simulink model "WMMSupportingForcesGP2020a"  (R2020a)
settings: Solver=ode23t  StartTime=0.0  StopTime=inf  FixedStep=.001  RelTol=1e-3  AbsTol=1e-3
InitFcn:
  | InitializeSimulationGP
  | SimulationParametersGP
values from neighbouring files (symbols this model uses):
  B11_r_B11C = [0.23805608; 0.13201777; 0]    [InitializeSimulationGP.m]
  B11_r_B11Tc1 = [L11; 0; 0]    [InitializeSimulationGP.m]
  B11_Rot_Tc1 = eye(3)    [InitializeSimulationGP.m]
  B11cI = [0.28426000 -0.06487287 0;         -0.06487287  0.54237481 0;                   0  0          0.67891020]    [InitializeSimulationGP.m]
  B12_r_B12C = [0.60504569; 0.27199376; 0.00002484]    [InitializeSimulationGP.m]
  B12_r_B12Tc2 = [L12;0;0]    [InitializeSimulationGP.m]
  B12_Rot_Tc2 = eye(3)    [InitializeSimulationGP.m]
  B12cI = [1.18803886 -2.36786418 0.00280315;          -2.36786418 6.31493281 0.00022322;           0.00280315 0.00022322 7.40915161]    [InitializeSimulationGP.m]
  B31_r_B31C = [0.35781210 0 0]    [InitializeSimulationGP.m]
  B31_Rot_B41 = eye(3)    [InitializeSimulationGP.m]
  B31cI = diag([0.03150902 0.90735702 0.90763033])    [InitializeSimulationGP.m]
  B32_r_B32C = [0.35781210 0 0]    [InitializeSimulationGP.m]
  B32_Rot_B42 = eye(3)    [InitializeSimulationGP.m]
  B32cI = diag([0.03150902 0.90735702 0.90763033])    [InitializeSimulationGP.m]
  B41_r_B41C = [0.55785997 0 0]    [InitializeSimulationGP.m]
  B41_r_B41Tc1 = [lc1;0;0]    [InitializeSimulationGP.m]
  B41cI = diag([0.00370720 0.55759812 0.55785997])    [InitializeSimulationGP.m]
  B42_r_B42C = [0.55785997 0 0]    [InitializeSimulationGP.m]
  B42_r_B42Tc2 = [lc2; 0; 0]    [InitializeSimulationGP.m]
  B42cI = diag([0.00370720 0.55759812 0.55785997])    [InitializeSimulationGP.m]
  B52_r_B52C = [0 0 0.56802906]    [InitializeSimulationGP.m]
  B52_r_B52P32 = [lc3; 0; 0]    [InitializeSimulationGP.m]
  B52_Rot_P32 = eye(3)    [InitializeSimulationGP.m]
  B52cI = diag([0.91789884, 0.91790043, 0.00091463])    [InitializeSimulationGP.m]
  Bc1_r_Bc1B11 = [L1; 0; 0]    [InitializeSimulationGP.m]
  Bc1_r_Bc1B31 = [0;0;0]    [InitializeSimulationGP.m]
  Bc1_r_Bc1C = [0.14178771; 0.16555780; 0]    [InitializeSimulationGP.m]
  Bc1_V = [0;0;0;0;0;0]    [InitializeSimulationGP.m]
  Bc1cI = [+5.892211080 +5.476111360 -0.000019630;          +5.476111360 +28.66965601 -0.000024550;          -0.000019630 -0.000024550 +29.78955950]    [InitializeSimulationGP.m]
  Bc2_r_Bc2B12 = [L2;0;0]    [InitializeSimulationGP.m]
  Bc2_r_Bc2B32 = [0;0;0]    [InitializeSimulationGP.m]
  Bc2_r_Bc2C = [0.54319901; 0.10543875; 0]    [InitializeSimulationGP.m]
  Bc2cI = [0.48071390 0.52924041 0;          0.52924041 5.80912352 0;              0      0          5.97255351]    [InitializeSimulationGP.m]
  BC_r_BCBM = [xCA; yCA; zCA]    [SimulationParametersGP.m]
  BC_Rot_BM = eye(3)    [SimulationParametersGP.m]
  BCI = diag([100 1200 1000])    [SimulationParametersGP.m]
  beta1 = atan2d(374.261,935)*pi/180    [InitializeSimulationGP.m]
  beta2 = atan2d(45.757,373.313)*pi/180    [InitializeSimulationGP.m]
  beta3 = atan2d(139.50,1132.19)*pi/180    [InitializeSimulationGP.m]
  beta4 = atan2d(88.061,296.198)*pi/180    [InitializeSimulationGP.m]
  betaGround = 1e6    (= 1000000)    [SimulationParametersGP.m]
  BFL = 0.05    [SimulationParametersGP.m]
  BFR = 0.05    [SimulationParametersGP.m]
  BM_r_BMBMp = [0;0;0]    [SimulationParametersGP.m]
  BM_Rot_BMp = [cos(gamma) -sin(gamma) 0; sin(gamma) cos(gamma) 0; 0 0 1]    [SimulationParametersGP.m]
  BMp_r_BMpBc1 = [0.185;0;0.205]    [InitializeSimulationGP.m]
  BMp_Rot_Bc1 = [cos(alpha1) -sin(alpha1)  0;                  0            0       -1;                sin(alpha1)  cos(alpha1)  0]    [InitializeSimulationGP.m]
  BRL = 0.05    [SimulationParametersGP.m]
  BRR = 0.05    [SimulationParametersGP.m]
  cc = 0.0    (= 0)    [SimulationParametersGP.m]
  D22F = [0;0;0;0;0;0]    [InitializeSimulationGP.m]
  dT = 0.01    [SimulationParametersGP.m]
  g0 = 9.8066    [SimulationParametersGP.m]
  ground_stiffness = 1e8    (= 100000000)    [SimulationParametersGP.m]
  l1 = 1.15-cc    (= 1.15)    [SimulationParametersGP.m]
  L1 = 1.0071227324212    (= 1.00712273242)    [InitializeSimulationGP.m]
  L11 = 0.37610632101293    (= 0.376106321013)    [InitializeSimulationGP.m]
  L12 = 0.30901132665325    (= 0.309011326653)    [InitializeSimulationGP.m]
  l2 = 1.15+cc    (= 1.15)    [SimulationParametersGP.m]
  L2 = 1.132185817991    (= 1.13218581799)    [InitializeSimulationGP.m]
  lc1 = 0.745    [InitializeSimulationGP.m]
  lc2 = 0.745    [InitializeSimulationGP.m]
  mB11 = 25.52660174    [InitializeSimulationGP.m]
  mB12 = 33.92850233    [InitializeSimulationGP.m]
  mB31 = 17.36281648    [InitializeSimulationGP.m]
  mB32 = 17.36281648    [InitializeSimulationGP.m]
  mB41 = 10.34519231    [InitializeSimulationGP.m]
  mB42 = 10.34519231    [InitializeSimulationGP.m]
  mB52 = 6.73059863    [InitializeSimulationGP.m]
  mBC = 2200    [SimulationParametersGP.m]
  mBc1 = 307.29601379    [InitializeSimulationGP.m]
  mBc2 = 54.58702836    [InitializeSimulationGP.m]
  mFL = 60    [SimulationParametersGP.m]
  mFR = 60    [SimulationParametersGP.m]
  mP22 = 9.26136143    [InitializeSimulationGP.m]
  mP32 = 570.18877059    [InitializeSimulationGP.m]
  mRR = 60    [SimulationParametersGP.m]
  mw = mFL    (= 60)    [SimulationParametersGP.m]
  P22_r_P22C = [0.62192523 0 0]    [InitializeSimulationGP.m]
  P22_Rot_B52 = eye(3)    [InitializeSimulationGP.m]
  P22cI = diag([0.00662754, 1.48387017, 1.48398069])    [InitializeSimulationGP.m]
  P32_r_P32C = [0.25466704; -0.13034397; -0.01302248]    [InitializeSimulationGP.m]
  P32_r_P32D22 = [0.40499744871392; -0.13130517281345; -0.013385243295654]    [InitializeSimulationGP.m]
  P32_Rot_D22 = [1 0 0;              0 0.9707729441837 0.23999977258512;              0 -0.23999977258512 0.9707729441837]    [InitializeSimulationGP.m]
  P32cI = [46.81220713 0.38607676 -0.00453819;          0.38607676 71.92201786 -1.14320993;          -0.00453819 -1.14320993 67.38128576]    [InitializeSimulationGP.m]
  R0FL = 0.35    [SimulationParametersGP.m]
  R0FR = 0.35    [SimulationParametersGP.m]
  R0RL = 0.35    [SimulationParametersGP.m]
  R0RR = 0.35    [SimulationParametersGP.m]
  Rw = R0FL    (= 0.35)    [SimulationParametersGP.m]
  Tc1_r_Tc1Bc2 = [0.098495302558553; 0.01838181329939; 0]    [InitializeSimulationGP.m]
  Tc1_Rot_Bc2 = [cos(alpha2) -sin(alpha2) 0;                sin(alpha2)  cos(alpha2) 0;                0            0           1]    [InitializeSimulationGP.m]
  Tc2_r_Tc2P22 = [-0.048858374920227;0.36587359346146;0.035276938723102]    [InitializeSimulationGP.m]
  Tc2_Rot_P22 = [0.95853460763586 -0.27664713597974  0.0683942111482;                0.28497614981675  0.93051946315663 -0.23004808784757;                0                 0.23999977258511  0.9707729441837]    [InitializeSimulationGP.m]
  Th1A = 10*pi/180    (= 0.174532925199)    [InitializeSimulationGP.m]
  Th1B = 20*pi/180    (= 0.349065850399)    [InitializeSimulationGP.m]
  Th1f = 1    [InitializeSimulationGP.m]
  Th2A = 15*pi/180    (= 0.261799387799)    [InitializeSimulationGP.m]
  Th2B = -70*pi/180    (= -1.2217304764)    [InitializeSimulationGP.m]
  Th2f = 2    [InitializeSimulationGP.m]
  w = wFL    (= 0.875)    [SimulationParametersGP.m]
  W_r_WBc1 = [0.185;0;0.205]    [InitializeSimulationGP.m]
  W_Rot_Bc1 = [cos(alpha1) -sin(alpha1)  0;                  0            0       -1;                sin(alpha1)  cos(alpha1)  0]    [InitializeSimulationGP.m]
  x10 = 0.83    [InitializeSimulationGP.m]
  x20 = 0.83    [InitializeSimulationGP.m]
  x3A = 0.2    [InitializeSimulationGP.m]
  x3B = 0.3    [InitializeSimulationGP.m]
  x3f = 1    [InitializeSimulationGP.m]
  xCA = 0.5    [SimulationParametersGP.m]
  xf = [1;0;0;0;0;0]    [InitializeSimulationGP.m]
  yCA = 0    [SimulationParametersGP.m]
  zC = 0.45    [SimulationParametersGP.m]
  zCA = .25    (= 0.25)    [SimulationParametersGP.m]
  ztau = [0;0;0;0;0;1]    [InitializeSimulationGP.m]
undefined symbols (not defined in the file or in its folder): alphaFL_meas, alphaFR_meas, alphaRL_meas, alphaRR_meas, B11_V, B11Ftot, B12_U_Tc2, B12_V, B12Ftot, B31_r_B31B41, B31_V, B31FTot, B32_r_B32B42, B32_U_B42, B32_V, B32FTot, B41_V, B41FTot, B42_Rot_Tc2, B42_U_Tc2, B42_V, B42FTot, B52_U_P32, B52_V, B52Ftot, Bc1Tot, Bc2_Rot_B12, Bc2_Rot_B32, Bc2_U_B12, Bc2_U_B32, Bc2_V, Bc2Tot, betaC_meas, D22_V, deltaFL_cmd, deltaFL_meas, deltaFR_cmd, deltaFR_meas, deltaRL_cmd, deltaRL_meas, deltaRR_cmd, deltaRR_meas, dOmegaFL_meas, dOmegaFR_meas, dOmegaRL_meas, dOmegaRR_meas, dPsi_meas, dq1, dq11, dq12, dq2, dq21, dq22, dx1, dx2, Floor, FTot_S1, FTot_S2P, FTot_S2R, FzFL ... (+63)
libraries: sm_lib x94, nesl_utility x63, simulink x5
(part 11 of 11)

== matlab function WMMSupportingForcesGP2020a/calc_wheel_velocities_and_sideslip_angles_from_meas/Hydraulic manipulator, calculation/AnalyticTotalForces/Structure 2 (Prismatic segment)/MATLAB Function2 ==
  data: B52V input; B52a input; B52w input; B52dw input; B52_Rot_W input; Wg parameter; YB52 output
function YB52  = thetaB52(B52V, B52a, B52w, B52dw, B52_Rot_W,  Wg)

vx = B52V(1);
vy = B52V(2);
vz = B52V(3);
ax = B52a(1);
ay = B52a(2);
az = B52a(3);
wx = B52w(1);
wy = B52w(2);
wz = B52w(3);
dwx = B52dw(1);
dwy = B52dw(2);
dwz = B52dw(3);
B52g = B52_Rot_W*Wg;
gx = B52g(1);
gy = B52g(2);
gz = B52g(3);

Y11 = ( ax + vz * wy - vy * wz  + gx);
t5 = (wy *  wy);
t6 = (wz * wz);
Y12 = -t5 - t6;
t7 = (wx * wy);
Y13 = (t7 - dwz);
t8 = (wx * wz);
Y14 = (t8 + dwy);
Y15 = 0;
Y16 = 0;
Y17 = 0;
Y18 = 0;
Y19 = 0;
Y110 = 0;
Y111 = 0;
Y112 = 0;
Y113 = 0;
Y21 = vx * wz - vz * wx + ay + gy;
Y22 = t7 + dwz;
t11 = wx * wx;
Y23 = -t11 - t6;
t12 = wy * wz;
Y24 = t12 - dwx;
Y25 = 0;
Y26 = 0;
Y27 = 0;
Y28 = 0;
Y29 = 0;
Y210 = 0;
Y211 = 0;
Y212 = 0;
Y213 = 0;
Y31 = -vx * wy + vy * wx + az + gz;
Y32 = t8 - dwy;
Y33 = t12 + dwx;
Y34 = -t11 - t5;
Y35 = 0;
Y36 = 0;
Y37 = 0;
Y38 = 0;
Y39 = 0;
Y310 = 0;
Y311 = 0;
Y312 = 0;
Y313 = 0;
Y41 = 0;
Y42 = 0;
Y43 = Y31;
Y44 = -Y21;
Y45 = 0;
Y46 = Y33;
Y47 = -Y24;
Y48 = Y32;
Y49 = -Y22;
Y410 = -t5 + t6;
Y411 = dwx;
Y412 = -t12;
Y413 = t12;
Y51 = 0;
Y52 = -Y31;
Y53 = 0;
Y54 = Y11;
Y55 = -Y32;
Y56 = 0;
Y57 = Y14;
Y58 = -Y33;
Y59 = t11 - t6;
Y510 = Y13;
Y511 = t8;
Y512 = dwy;
Y513 = -t8;
Y61 = 0;
Y62 = Y21;
Y63 = -Y11;
Y64 = 0;
Y65 = Y22;
Y66 = -Y13;
Y67 = 0;
Y68 = t5 - t11;
Y69 = Y24;
Y610 = -Y14;
Y611 = -t7;
Y612 = t7;
Y613 = dwz;

YB52 = [Y11 Y12 Y13 Y14 Y15 Y16 Y17 Y18 Y19 Y110 Y111 Y112 Y113;...
        Y21 Y22 Y23 Y24 Y25 Y26 Y27 Y28 Y29 Y210 Y211 Y212 Y213;...
        Y31 Y32 Y33 Y34 Y35 Y36 Y37 Y38 Y39 Y310 Y311 Y312 Y313;...
        Y41 Y42 Y43 Y44 Y45 Y46 Y47 Y48 Y49 Y410 Y411 Y412 Y413;...
        Y51 Y52 Y53 Y54 Y55 Y56 Y57 Y58 Y59 Y510 Y511 Y512 Y513;...
        Y61 Y62 Y63 Y64 Y65 Y66 Y67 Y68 Y69 Y610 Y611 Y612 Y613];

== matlab function WMMSupportingForcesGP2020a/calc_wheel_velocities_and_sideslip_angles_from_meas/Hydraulic manipulator, calculation/AnalyticVelocities/Structure 2 (Revolute segment)/RotMatsS2R/B42_Rot_Tc2 ==
  data: q22 input; B42_Rot_Tc2 output
function B42_Rot_Tc2 = B42_Rot_Tc2(q22)

B42_Rot_Tc2 = [+cos(q22) -sin(q22) 0;...
               +sin(q22) +cos(q22) 0;...
                   0        0      1];

== matlab function WMMSupportingForcesGP2020a/calc_wheel_velocities_and_sideslip_angles_from_meas/Hydraulic manipulator, calculation/AnalyticTotalForces/Structure 2 (Prismatic segment)/MATLAB Function3 ==
  data: thetaP32 output; P32_r_P32C parameter; mP32 parameter; P32cI parameter
function thetaP32 = thetaP32(P32_r_P32C, mP32, P32cI)

rx = P32_r_P32C(1);
ry = P32_r_P32C(2);
rz = P32_r_P32C(3);

Ixx = P32cI(1,1);
Iyy = P32cI(2,2);
Izz = P32cI(3,3);
Iyz = P32cI(2,3);
Ixz = P32cI(1,3);
Ixy = P32cI(1,2);

t1 = rx*rx;
t2 = ry*ry;
t3 = rz*rz;
t4 = rx*mP32;

thetaP32 = [mP32; rx*mP32; ry*mP32; rz*mP32; t1*mP32; t2*mP32; t3*mP32; t4*ry - Ixy; t4*rz - Ixz; mP32*ry*rz - Iyz; Ixx; Iyy; Izz];

== matlab function WMMSupportingForcesGP2020a/calc_wheel_velocities_and_sideslip_angles_from_meas/Hydraulic manipulator, calculation/AnalyticTotalForces/Structure 2 (Prismatic segment)/MATLAB Function7 ==
  data: P22V input; P22a input; P22w input; P22dw input; P22_Rot_W input; Wg parameter; YP22 output
function YP22  = thetaP22(P22V, P22a, P22w, P22dw, P22_Rot_W,  Wg)

vx = P22V(1);
vy = P22V(2);
vz = P22V(3);
ax = P22a(1);
ay = P22a(2);
az = P22a(3);
wx = P22w(1);
wy = P22w(2);
wz = P22w(3);
dwx = P22dw(1);
dwy = P22dw(2);
dwz = P22dw(3);
P22g = P22_Rot_W*Wg;
gx = P22g(1);
gy = P22g(2);
gz = P22g(3);

Y11 = ( ax + vz * wy - vy * wz  + gx);
t5 = (wy *  wy);
t6 = (wz * wz);
Y12 = -t5 - t6;
t7 = (wx * wy);
Y13 = (t7 - dwz);
t8 = (wx * wz);
Y14 = (t8 + dwy);
Y15 = 0;
Y16 = 0;
Y17 = 0;
Y18 = 0;
Y19 = 0;
Y110 = 0;
Y111 = 0;
Y112 = 0;
Y113 = 0;
Y21 = vx * wz - vz * wx + ay + gy;
Y22 = t7 + dwz;
t11 = wx * wx;
Y23 = -t11 - t6;
t12 = wy * wz;
Y24 = t12 - dwx;
Y25 = 0;
Y26 = 0;
Y27 = 0;
Y28 = 0;
Y29 = 0;
Y210 = 0;
Y211 = 0;
Y212 = 0;
Y213 = 0;
Y31 = -vx * wy + vy * wx + az + gz;
Y32 = t8 - dwy;
Y33 = t12 + dwx;
Y34 = -t11 - t5;
Y35 = 0;
Y36 = 0;
Y37 = 0;
Y38 = 0;
Y39 = 0;
Y310 = 0;
Y311 = 0;
Y312 = 0;
Y313 = 0;
Y41 = 0;
Y42 = 0;
Y43 = Y31;
Y44 = -Y21;
Y45 = 0;
Y46 = Y33;
Y47 = -Y24;
Y48 = Y32;
Y49 = -Y22;
Y410 = -t5 + t6;
Y411 = dwx;
Y412 = -t12;
Y413 = t12;
Y51 = 0;
Y52 = -Y31;
Y53 = 0;
Y54 = Y11;
Y55 = -Y32;
Y56 = 0;
Y57 = Y14;
Y58 = -Y33;
Y59 = t11 - t6;
Y510 = Y13;
Y511 = t8;
Y512 = dwy;
Y513 = -t8;
Y61 = 0;
Y62 = Y21;
Y63 = -Y11;
Y64 = 0;
Y65 = Y22;
Y66 = -Y13;
Y67 = 0;
Y68 = t5 - t11;
Y69 = Y24;
Y610 = -Y14;
Y611 = -t7;
Y612 = t7;
Y613 = dwz;

YP22 = [Y11 Y12 Y13 Y14 Y15 Y16 Y17 Y18 Y19 Y110 Y111 Y112 Y113;...
        Y21 Y22 Y23 Y24 Y25 Y26 Y27 Y28 Y29 Y210 Y211 Y212 Y213;...
        Y31 Y32 Y33 Y34 Y35 Y36 Y37 Y38 Y39 Y310 Y311 Y312 Y313;...
        Y41 Y42 Y43 Y44 Y45 Y46 Y47 Y48 Y49 Y410 Y411 Y412 Y413;...
        Y51 Y52 Y53 Y54 Y55 Y56 Y57 Y58 Y59 Y510 Y511 Y512 Y513;...
        Y61 Y62 Y63 Y64 Y65 Y66 Y67 Y68 Y69 Y610 Y611 Y612 Y613];

== matlab function WMMSupportingForcesGP2020a/calc_wheel_velocities_and_sideslip_angles_from_meas/Hydraulic manipulator, calculation/AnalyticVelocities/Structure 2 (Revolute segment)/GeomPropS2R/Subsystem4/q21AngularVelocity ==
  data: x2 input; dx2 input; q21 input; dq21 output; L2 parameter; x20 parameter
function dq21 = dq21(x2, dx2, q21, L2, x20)

dq21 = -((x2+x20)-L2*cos(q21))/((x2+x20)*L2*sin(q21))*dx2;

== matlab function WMMSupportingForcesGP2020a/calc_wheel_velocities_and_sideslip_angles_from_meas/Hydraulic manipulator, calculation/AnalyticVelocities/Structure 2 (Revolute segment)/GeomPropS2R/Subsystem5/q22AngularVelocity ==
  data: x2 input; dx2 input; q22 input; dq22 output; L12 parameter; x20 parameter
function dq22 = dq22(x2, dx2, q22, L12, x20)

dq22 = -((x2+x20)-L12*cos(q22))/((x2+x20)*L12*sin(q22))*dx2;

== matlab function WMMSupportingForcesGP2020a/calc_wheel_velocities_and_sideslip_angles_from_meas/Hydraulic manipulator, calculation/AnalyticVelocities/Structure 2 (Revolute segment)/GeomPropS2R/TiltPistonVelocity/TiltPistonVelocity ==
  data: x2 input; q2 input; dq2 input; dx2 output; L2 parameter; L12 parameter; x20 parameter
function dx2 = dx2(x2, q2, dq2, L2, L12, x20)

dx2 = -(L2*L12*sin(q2))/(x2+x20)*dq2;

== matlab function WMMSupportingForcesGP2020a/calc_wheel_velocities_and_sideslip_angles_from_meas/Hydraulic manipulator, calculation/AnalyticTotalForces/Structure 2 (Prismatic segment)/MATLAB Function4 ==
  data: P32V input; P32a input; P32w input; P32dw input; P32_Rot_W input; Wg parameter; YP32 output
function YP32  = thetaP32(P32V, P32a, P32w, P32dw, P32_Rot_W,  Wg)

vx = P32V(1);
vy = P32V(2);
vz = P32V(3);
ax = P32a(1);
ay = P32a(2);
az = P32a(3);
wx = P32w(1);
wy = P32w(2);
wz = P32w(3);
dwx = P32dw(1);
dwy = P32dw(2);
dwz = P32dw(3);
P32g = P32_Rot_W*Wg;
gx = P32g(1);
gy = P32g(2);
gz = P32g(3);

Y11 = ( ax + vz * wy - vy * wz  + gx);
t5 = (wy *  wy);
t6 = (wz * wz);
Y12 = -t5 - t6;
t7 = (wx * wy);
Y13 = (t7 - dwz);
t8 = (wx * wz);
Y14 = (t8 + dwy);
Y15 = 0;
Y16 = 0;
Y17 = 0;
Y18 = 0;
Y19 = 0;
Y110 = 0;
Y111 = 0;
Y112 = 0;
Y113 = 0;
Y21 = vx * wz - vz * wx + ay + gy;
Y22 = t7 + dwz;
t11 = wx * wx;
Y23 = -t11 - t6;
t12 = wy * wz;
Y24 = t12 - dwx;
Y25 = 0;
Y26 = 0;
Y27 = 0;
Y28 = 0;
Y29 = 0;
Y210 = 0;
Y211 = 0;
Y212 = 0;
Y213 = 0;
Y31 = -vx * wy + vy * wx + az + gz;
Y32 = t8 - dwy;
Y33 = t12 + dwx;
Y34 = -t11 - t5;
Y35 = 0;
Y36 = 0;
Y37 = 0;
Y38 = 0;
Y39 = 0;
Y310 = 0;
Y311 = 0;
Y312 = 0;
Y313 = 0;
Y41 = 0;
Y42 = 0;
Y43 = Y31;
Y44 = -Y21;
Y45 = 0;
Y46 = Y33;
Y47 = -Y24;
Y48 = Y32;
Y49 = -Y22;
Y410 = -t5 + t6;
Y411 = dwx;
Y412 = -t12;
Y413 = t12;
Y51 = 0;
Y52 = -Y31;
Y53 = 0;
Y54 = Y11;
Y55 = -Y32;
Y56 = 0;
Y57 = Y14;
Y58 = -Y33;
Y59 = t11 - t6;
Y510 = Y13;
Y511 = t8;
Y512 = dwy;
Y513 = -t8;
Y61 = 0;
Y62 = Y21;
Y63 = -Y11;
Y64 = 0;
Y65 = Y22;
Y66 = -Y13;
Y67 = 0;
Y68 = t5 - t11;
Y69 = Y24;
Y610 = -Y14;
Y611 = -t7;
Y612 = t7;
Y613 = dwz;

YP32 = [Y11 Y12 Y13 Y14 Y15 Y16 Y17 Y18 Y19 Y110 Y111 Y112 Y113;...
        Y21 Y22 Y23 Y24 Y25 Y26 Y27 Y28 Y29 Y210 Y211 Y212 Y213;...
        Y31 Y32 Y33 Y34 Y35 Y36 Y37 Y38 Y39 Y310 Y311 Y312 Y313;...
        Y41 Y42 Y43 Y44 Y45 Y46 Y47 Y48 Y49 Y410 Y411 Y412 Y413;...
        Y51 Y52 Y53 Y54 Y55 Y56 Y57 Y58 Y59 Y510 Y511 Y512 Y513;...
        Y61 Y62 Y63 Y64 Y65 Y66 Y67 Y68 Y69 Y610 Y611 Y612 Y613];

== matlab function WMMSupportingForcesGP2020a/calc_wheel_velocities_and_sideslip_angles_from_meas/Hydraulic manipulator, calculation/AnalyticVelocities/Structure 2 (Revolute segment)/RotMatsS2R/Bc2_Rot_B12 ==
  data: q2 input; Bc2_Rot_B12 output
function Bc2_Rot_B12 = Bc2_Rot_B12(q2)

Bc2_Rot_B12 = [+cos(q2) -sin(q2) 0;...
               +sin(q2) +cos(q2) 0;...
                  0        0     1];

== matlab function WMMSupportingForcesGP2020a/calc_wheel_velocities_and_sideslip_angles_from_meas/Hydraulic manipulator, calculation/AnalyticVelocities/Structure 2 (Revolute segment)/RotMatsS2R/Bc2_Rot_B32 ==
  data: q21 input; Bc2_Rot_B32 output

function Bc2_Rot_B32 = Bc2_Rot_B32(q21)

Bc2_Rot_B32 = [+cos(q21) -sin(q21) 0;...
               +sin(q21) +cos(q21) 0;...
                   0         0     1];

== matlab function WMMSupportingForcesGP2020a/calc_wheel_velocities_and_sideslip_angles_from_meas/Hydraulic manipulator, calculation/AnalyticVelocities/Structure 2 (Revolute segment)/UMatS2R/B12_U_Tc2 ==
  data: B12_r_B12Tc2 input; B12_U_Tc2 output; B12_Rot_Tc2 input
function B12_U_Tc2 = B12_U_Tc2(B12_r_B12Tc2, B12_Rot_Tc2)

B12_U_Tc2 = [B12_Rot_Tc2,                    zeros(3);...
             dual(B12_r_B12Tc2)*B12_Rot_Tc2, B12_Rot_Tc2];
   
end
   
function dual_r = dual(ArAB)

dual_r = [0,  -ArAB(3), ArAB(2);...
          ArAB(3), 0, -ArAB(1);...
          -ArAB(2), ArAB(1), 0];

end

== matlab function WMMSupportingForcesGP2020a/calc_wheel_velocities_and_sideslip_angles_from_meas/Hydraulic manipulator, calculation/AnalyticVelocities/Structure 2 (Revolute segment)/UMatS2R/B32_U_B42 ==
  data: B32_r_B32B42 input; B32_U_B42 output; B32_Rot_B42 input
function B32_U_B42 = B32_U_B42(B32_r_B32B42, B32_Rot_B42)

B32_U_B42 = [B32_Rot_B42,                    zeros(3);...
             dual(B32_r_B32B42)*B32_Rot_B42, B32_Rot_B42];
   
end
   
function dual_r = dual(ArAB)

dual_r = [0,  -ArAB(3), ArAB(2);...
          ArAB(3), 0, -ArAB(1);...
          -ArAB(2), ArAB(1), 0];

end

== matlab function WMMSupportingForcesGP2020a/calc_wheel_velocities_and_sideslip_angles_from_meas/Hydraulic manipulator, calculation/AnalyticVelocities/Structure 2 (Revolute segment)/UMatS2R/B42_U_Tc2 ==
  data: B42_r_B42Tc2 input; B42_U_Tc2 output; B42_Rot_Tc2 input
function B42_U_Tc2 = B42_U_Tc2(B42_r_B42Tc2, B42_Rot_Tc2)

B42_U_Tc2 = [B42_Rot_Tc2,                    zeros(3);...
             dual(B42_r_B42Tc2)*B42_Rot_Tc2, B42_Rot_Tc2];
   
end
   
function dual_r = dual(ArAB)

dual_r = [0,  -ArAB(3), ArAB(2);...
          ArAB(3), 0, -ArAB(1);...
          -ArAB(2), ArAB(1), 0];

end

== matlab function WMMSupportingForcesGP2020a/calc_wheel_velocities_and_sideslip_angles_from_meas/Hydraulic manipulator, calculation/AnalyticVelocities/Structure 2 (Revolute segment)/UMatS2R/Bc2_U_B12 ==
  data: Bc2_r_Bc2B12 input; Bc2_U_B12 output; Bc2_Rot_B12 input
function Bc2_U_B12 = Bc2_U_B12(Bc2_r_Bc2B12, Bc2_Rot_B12)

Bc2_U_B12 = [Bc2_Rot_B12,                    zeros(3);...
             dual(Bc2_r_Bc2B12)*Bc2_Rot_B12, Bc2_Rot_B12];
   
end
   
function dual_r = dual(ArAB)

dual_r = [0,  -ArAB(3), ArAB(2);...
          ArAB(3), 0, -ArAB(1);...
          -ArAB(2), ArAB(1), 0];

end

== matlab function WMMSupportingForcesGP2020a/calc_wheel_velocities_and_sideslip_angles_from_meas/Hydraulic manipulator, calculation/AnalyticVelocities/Structure 2 (Revolute segment)/UMatS2R/Bc2_U_B32 ==
  data: Bc2_r_Bc2B32 input; Bc2_U_B32 output; Bc2_Rot_B32 input
function Bc2_U_B32 = Bc2_U_B32(Bc2_r_Bc2B32, Bc2_Rot_B32)

Bc2_U_B32 = [Bc2_Rot_B32,                    zeros(3);...
             dual(Bc2_r_Bc2B32)*Bc2_Rot_B32, Bc2_Rot_B32];
   
end
   
function dual_r = dual(ArAB)

dual_r = [0,  -ArAB(3), ArAB(2);...
          ArAB(3), 0, -ArAB(1);...
          -ArAB(2), ArAB(1), 0];

end

== matlab function WMMSupportingForcesGP2020a/calc_wheel_velocities_and_sideslip_angles_from_meas/Hydraulic manipulator, calculation/AnalyticVelocities/Structure 2 (Revolute segment)/UMatS2R/Tc2_U_P22 ==
  data: Tc2_r_Tc2P22 input; Tc2_U_P22 output; Tc2_Rot_P22 input
function Tc2_U_P22 = Tc2_U_P22(Tc2_r_Tc2P22, Tc2_Rot_P22)

Tc2_U_P22 = [Tc2_Rot_P22,                    zeros(3);...
             dual(Tc2_r_Tc2P22)*Tc2_Rot_P22, Tc2_Rot_P22];
   
end
   
function dual_r = dual(ArAB)

dual_r = [0,  -ArAB(3), ArAB(2);...
          ArAB(3), 0, -ArAB(1);...
          -ArAB(2), ArAB(1), 0];

end

== matlab function WMMSupportingForcesGP2020a/calc_wheel_velocities_and_sideslip_angles_from_meas/BM_U_BMp ==
  data: BM_r_BMBMp input; BM_U_BMp output; BM_Rot_BMp input
function BM_U_BMp = BM_U_BMp(BM_r_BMBMp, BM_Rot_BMp)

BM_U_BMp = [BM_Rot_BMp,                    zeros(3);...
             dual(BM_r_BMBMp)*BM_Rot_BMp, BM_Rot_BMp];
   
end
   
function dual_r = dual(ArAB)

dual_r = [0,  -ArAB(3), ArAB(2);...
          ArAB(3), 0, -ArAB(1);...
          -ArAB(2), ArAB(1), 0];

end

== matlab function WMMSupportingForcesGP2020a/calc_wheel_velocities_and_sideslip_angles_from_meas/Hydraulic manipulator, calculation/AnalyticTotalForces/Structure 2 (Revolute segment)/MATLAB Function1 ==
  data: Bc2V input; Bc2a input; Bc2w input; Bc2dw input; Bc2_Rot_W input; Wg parameter; YBc2 output
function YBc2  = thetaBc2(Bc2V, Bc2a, Bc2w, Bc2dw, Bc2_Rot_W,  Wg)

vx = Bc2V(1);
vy = Bc2V(2);
vz = Bc2V(3);
ax = Bc2a(1);
ay = Bc2a(2);
az = Bc2a(3);
wx = Bc2w(1);
wy = Bc2w(2);
wz = Bc2w(3);
dwx = Bc2dw(1);
dwy = Bc2dw(2);
dwz = Bc2dw(3);
Bc2g = Bc2_Rot_W*Wg;
gx = Bc2g(1);
gy = Bc2g(2);
gz = Bc2g(3);

Y11 = ( ax + vz * wy - vy * wz  + gx);
t5 = (wy *  wy);
t6 = (wz * wz);
Y12 = -t5 - t6;
t7 = (wx * wy);
Y13 = (t7 - dwz);
t8 = (wx * wz);
Y14 = (t8 + dwy);
Y15 = 0;
Y16 = 0;
Y17 = 0;
Y18 = 0;
Y19 = 0;
Y110 = 0;
Y111 = 0;
Y112 = 0;
Y113 = 0;
Y21 = vx * wz - vz * wx + ay + gy;
Y22 = t7 + dwz;
t11 = wx * wx;
Y23 = -t11 - t6;
t12 = wy * wz;
Y24 = t12 - dwx;
Y25 = 0;
Y26 = 0;
Y27 = 0;
Y28 = 0;
Y29 = 0;
Y210 = 0;
Y211 = 0;
Y212 = 0;
Y213 = 0;
Y31 = -vx * wy + vy * wx + az + gz;
Y32 = t8 - dwy;
Y33 = t12 + dwx;
Y34 = -t11 - t5;
Y35 = 0;
Y36 = 0;
Y37 = 0;
Y38 = 0;
Y39 = 0;
Y310 = 0;
Y311 = 0;
Y312 = 0;
Y313 = 0;
Y41 = 0;
Y42 = 0;
Y43 = Y31;
Y44 = -Y21;
Y45 = 0;
Y46 = Y33;
Y47 = -Y24;
Y48 = Y32;
Y49 = -Y22;
Y410 = -t5 + t6;
Y411 = dwx;
Y412 = -t12;
Y413 = t12;
Y51 = 0;
Y52 = -Y31;
Y53 = 0;
Y54 = Y11;
Y55 = -Y32;
Y56 = 0;
Y57 = Y14;
Y58 = -Y33;
Y59 = t11 - t6;
Y510 = Y13;
Y511 = t8;
Y512 = dwy;
Y513 = -t8;
Y61 = 0;
Y62 = Y21;
Y63 = -Y11;
Y64 = 0;
Y65 = Y22;
Y66 = -Y13;
Y67 = 0;
Y68 = t5 - t11;
Y69 = Y24;
Y610 = -Y14;
Y611 = -t7;
Y612 = t7;
Y613 = dwz;

YBc2 = [Y11 Y12 Y13 Y14 Y15 Y16 Y17 Y18 Y19 Y110 Y111 Y112 Y113;...
        Y21 Y22 Y23 Y24 Y25 Y26 Y27 Y28 Y29 Y210 Y211 Y212 Y213;...
        Y31 Y32 Y33 Y34 Y35 Y36 Y37 Y38 Y39 Y310 Y311 Y312 Y313;...
        Y41 Y42 Y43 Y44 Y45 Y46 Y47 Y48 Y49 Y410 Y411 Y412 Y413;...
        Y51 Y52 Y53 Y54 Y55 Y56 Y57 Y58 Y59 Y510 Y511 Y512 Y513;...
        Y61 Y62 Y63 Y64 Y65 Y66 Y67 Y68 Y69 Y610 Y611 Y612 Y613];

== matlab function WMMSupportingForcesGP2020a/calc_wheel_velocities_and_sideslip_angles_from_meas/BMp_U_Bc1 ==
  data: BMp_r_BMpBc1 input; BMp_U_Bc1 output; BMp_Rot_Bc1 input
function BMp_U_Bc1 = BMp_U_Bc1(BMp_r_BMpBc1, BMp_Rot_Bc1)

BMp_U_Bc1 = [BMp_Rot_Bc1,                    zeros(3);...
             dual(BMp_r_BMpBc1)*BMp_Rot_Bc1, BMp_Rot_Bc1];
   
end
   
function dual_r = dual(ArAB)

dual_r = [0,  -ArAB(3), ArAB(2);...
          ArAB(3), 0, -ArAB(1);...
          -ArAB(2), ArAB(1), 0];

end

== matlab function WMMSupportingForcesGP2020a/calc_wheel_velocities_and_sideslip_angles_from_meas/Hydraulic manipulator, calculation/AnalyticVelocities/Structure 2 (Prismatic segment)/UMatsS2P/P32_U_D22 ==
  data: P32_r_P32D22 input; P32_U_D22 output; P32_Rot_D22 input
function P32_U_D22 = P32_U_D22(P32_r_P32D22, P32_Rot_D22)

P32_U_D22 = [P32_Rot_D22,                    zeros(3);...
              dual(P32_r_P32D22)*P32_Rot_D22, P32_Rot_D22];
   
end
   
function dual_r = dual(ArAB)

dual_r = [0,  -ArAB(3), ArAB(2);...
          ArAB(3), 0, -ArAB(1);...
          -ArAB(2), ArAB(1), 0];

end

== matlab function WMMSupportingForcesGP2020a/MATLAB Function ==
  data: GRotBC input; TFL_fz output; l1 parameter; l2 parameter; mw parameter; Rw parameter; zC parameter; mBC parameter; w parameter; BMF input; xCA parameter; yCA parameter; zCA parameter; BCvX input; BCvY input; dPsi input; BCaX input; BCaY input; ddPsi input; g0 parameter; BCI parameter size=[3,3]
function TFL_fz = fcn(GRotBC, l1, l2, mw, Rw, zC, mBC, w, BMF, xCA, yCA, zCA, BCvX, BCvY, dPsi, BCaX, BCaY, ddPsi, g0, BCI)


r31 = GRotBC(3,1); r32 = GRotBC(3,2); r33 = GRotBC(3,3);

BMfx = BMF(1);     BMfy = BMF(2);     BMfz = BMF(3);
BMmx = BMF(4);     BMmy = BMF(5);     

BCIxz = BCI(1,3);  BCIyz = BCI(2,3);

zetaFL1 = g0*(mBC/2 * l1/(l1+l2) + mw)*r33 - g0*(mw*Rw + 0.25*mBC*zC)/w*r32 -...
          2*g0*(mw*Rw + 0.25*mBC*zC)/(l1+l2)*r31;
zetaFL2 = 0.5*(zCA + zC)/(l1+l2)*BMfx;
zetaFL3 = 0.25*(zCA + zC)/w*BMfy;
zetaFL4 = -0.5*((l1+xCA)/(l1+l2) + 0.5*yCA/w)*BMfz;
zetaFL5 = -BMmx/4/w;
zetaFL6 = 0.5*BMmy/(l1+l2);
zetaFL7 = -0.5*mBC*zC/(l1+l2)*BCaX;
zetaFL8 = -0.25*mBC*zC/w*BCaY;
zetaFL9 = 0.5*mBC*zC*(-BCvX/(2*w) + BCvY/(l1+l2))*dPsi;
zetaFL10 = -0.5*(BCIxz/(l1+l2) + BCIyz/(2*w))*dPsi*dPsi;
zetaFL11 = -0.5*(BCIyz/(l1+l2) - BCIxz/(2*w))*ddPsi;

TFL_fz = zetaFL1 + zetaFL2 + zetaFL3+ zetaFL4 + zetaFL5 + zetaFL6 + ...
         zetaFL7 + zetaFL8 + zetaFL9 + zetaFL10 + zetaFL11;

== matlab function WMMSupportingForcesGP2020a/calc_wheel_velocities_and_sideslip_angles_from_meas/MATLAB Function1 ==
  data: Theta input; GRotBC output; Phi input; Psi input
function GRotBC = GRotBC(Theta, Phi, Psi)

cTh = cos(Theta);
sTh = sin(Theta);
cPhi = cos(Phi);
sPhi = sin(Phi);
cPsi = cos(Psi);
sPsi = sin(Psi);

GRotBC = [cTh*cPsi+sTh*sPhi*sPsi cPsi*sTh*sPhi - cTh*sPsi cPhi*sTh;...
          cPhi*sPsi cPhi*cPsi -sPhi;...
          -cPsi*sTh + cTh*sPhi*sPsi cTh*cPsi*sPhi+sTh*sPsi cTh*cPhi];

== matlab function WMMSupportingForcesGP2020a/MATLAB Function2 ==
  data: GRotBC input; TFR_fz output; l1 parameter; l2 parameter; mw parameter; Rw parameter; zC parameter; mBC parameter; w parameter; BMF input; xCA parameter; yCA parameter; zCA parameter; BCvX input; BCvY input; dPsi input; BCaX input; BCaY input; ddPsi input; g0 parameter; BCI parameter size=[3,3]
function TFR_fz = fcn(GRotBC, l1, l2, mw, Rw, zC, mBC, w, BMF, xCA, yCA, zCA, BCvX, BCvY, dPsi, BCaX, BCaY, ddPsi, g0, BCI)


r31 = GRotBC(3,1); r32 = GRotBC(3,2); r33 = GRotBC(3,3);

BMfx = BMF(1);     BMfy = BMF(2);     BMfz = BMF(3);
BMmx = BMF(4);     BMmy = BMF(5);     

BCIxz = BCI(1,3);  BCIyz = BCI(2,3);

zetaFR1 = g0*(mBC/2 * l1/(l1+l2) + mw)*r33 + g0*(mw*Rw + 0.25*mBC*zC)/w*r32 -...
          2*g0*(mw*Rw + 0.25*mBC*zC)/(l1+l2)*r31;
zetaFR2 = 0.5*(zCA + zC)/(l1+l2)*BMfx;
zetaFR3 = -0.25*(zCA + zC)/w*BMfy;
zetaFR4 = -0.5*((l1+xCA)/(l1+l2) - 0.5*yCA/w)*BMfz;
zetaFR5 = BMmx/4/w;
zetaFR6 = 0.5*BMmy/(l1+l2);
zetaFR7 = -0.5*mBC*zC/(l1+l2)*BCaX;
zetaFR8 = 0.25*mBC*zC/w*BCaY;
zetaFR9 = 0.5*mBC*zC*(BCvX/(2*w) + BCvY/(l1+l2))*dPsi;
zetaFR10 = -0.5*(BCIxz/(l1+l2) - BCIyz/(2*w))*dPsi*dPsi;
zetaFR11 = -0.5*(BCIyz/(l1+l2) + BCIxz/(2*w))*ddPsi;

TFR_fz = zetaFR1 + zetaFR2 + zetaFR3+ zetaFR4 + zetaFR5 + zetaFR6 + ...
         zetaFR7 + zetaFR8 + zetaFR9 + zetaFR10 + zetaFR11;

== matlab function WMMSupportingForcesGP2020a/MATLAB Function1 ==
  data: GRotBC input; TRR_fz output; l1 parameter; l2 parameter; mw parameter; Rw parameter; zC parameter; mBC parameter; w parameter; BMF input; xCA parameter; yCA parameter; zCA parameter; BCvX input; BCvY input; dPsi input; BCaX input; BCaY input; ddPsi input; g0 parameter; BCI parameter size=[3,3]
function TRR_fz = fcn(GRotBC, l1, l2, mw, Rw, zC, mBC, w, BMF, xCA, yCA, zCA, BCvX, BCvY, dPsi, BCaX, BCaY, ddPsi, g0, BCI)


r31 = GRotBC(3,1); r32 = GRotBC(3,2); r33 = GRotBC(3,3);

BMfx = BMF(1);     BMfy = BMF(2);     BMfz = BMF(3);
BMmx = BMF(4);     BMmy = BMF(5);     

BCIxz = BCI(1,3);  BCIyz = BCI(2,3);

zetaRR1 = g0*(mBC/2 * l2/(l1+l2) + mw)*r33 + g0*(mw*Rw + 0.25*mBC*zC)/w*r32 +...
          2*g0*(mw*Rw + 0.25*mBC*zC)/(l1+l2)*r31;
zetaRR2 = -0.5*(zCA + zC)/(l1+l2)*BMfx;
zetaRR3 = -0.25*(zCA + zC)/w*BMfy;
zetaRR4 = -0.5*((l2-xCA)/(l1+l2) - 0.5*yCA/w)*BMfz;
zetaRR5 = BMmx/4/w;
zetaRR6 = -0.5*BMmy/(l1+l2);
zetaRR7 = 0.5*mBC*zC/(l1+l2)*BCaX;
zetaRR8 = 0.25*mBC*zC/w*BCaY;
zetaRR9 = 0.5*mBC*zC*(BCvX/(2*w) - BCvY/(l1+l2))*dPsi;
zetaRR10 = 0.5*(BCIxz/(l1+l2) + BCIyz/(2*w))*dPsi*dPsi;
zetaRR11 = 0.5*(BCIyz/(l1+l2) - BCIxz/(2*w))*ddPsi;

TRR_fz = zetaRR1 + zetaRR2 + zetaRR3+ zetaRR4 + zetaRR5 + zetaRR6 + ...
         zetaRR7 + zetaRR8 + zetaRR9 + zetaRR10 + zetaRR11;

== matlab function WMMSupportingForcesGP2020a/calc_wheel_velocities_and_sideslip_angles_from_meas/BC_U_BM ==
  data: BC_r_BCBM input; BC_U_BM output; BC_Rot_BM input
function BC_U_BM = BC_U_BM(BC_r_BCBM, BC_Rot_BM)

BC_U_BM = [BC_Rot_BM,                    zeros(3);...
           dual(BC_r_BCBM)*BC_Rot_BM, BC_Rot_BM];
   
end
   
function dual_r = dual(ArAB)

dual_r = [0,  -ArAB(3), ArAB(2);...
          ArAB(3), 0, -ArAB(1);...
          -ArAB(2), ArAB(1), 0];

end

== matlab function WMMSupportingForcesGP2020a/calc_wheel_velocities_and_sideslip_angles_from_meas/BM_Rot_BMp ==
  data: BM_Rot_BMp output; gamma parameter
function BM_Rot_BMp = BM_Rot_BMp(gamma)

BM_Rot_BMp = [cos(gamma) -sin(gamma) 0; sin(gamma) cos(gamma) 0; 0 0 1];

== matlab function WMMSupportingForcesGP2020a/calc_wheel_velocities_and_sideslip_angles_from_meas/Hydraulic manipulator, calculation/AnalyticTotalForces/Structure 2 (Revolute segment)/MATLAB Function7 ==
  data: B42V input; B42a input; B42w input; B42dw input; B42_Rot_W input; Wg parameter; YB42 output
function YB42  = thetaB42(B42V, B42a, B42w, B42dw, B42_Rot_W,  Wg)

vx = B42V(1);
vy = B42V(2);
vz = B42V(3);
ax = B42a(1);
ay = B42a(2);
az = B42a(3);
wx = B42w(1);
wy = B42w(2);
wz = B42w(3);
dwx = B42dw(1);
dwy = B42dw(2);
dwz = B42dw(3);
B42g = B42_Rot_W*Wg;
gx = B42g(1);
gy = B42g(2);
gz = B42g(3);

Y11 = ( ax + vz * wy - vy * wz  + gx);
t5 = (wy *  wy);
t6 = (wz * wz);
Y12 = -t5 - t6;
t7 = (wx * wy);
Y13 = (t7 - dwz);
t8 = (wx * wz);
Y14 = (t8 + dwy);
Y15 = 0;
Y16 = 0;
Y17 = 0;
Y18 = 0;
Y19 = 0;
Y110 = 0;
Y111 = 0;
Y112 = 0;
Y113 = 0;
Y21 = vx * wz - vz * wx + ay + gy;
Y22 = t7 + dwz;
t11 = wx * wx;
Y23 = -t11 - t6;
t12 = wy * wz;
Y24 = t12 - dwx;
Y25 = 0;
Y26 = 0;
Y27 = 0;
Y28 = 0;
Y29 = 0;
Y210 = 0;
Y211 = 0;
Y212 = 0;
Y213 = 0;
Y31 = -vx * wy + vy * wx + az + gz;
Y32 = t8 - dwy;
Y33 = t12 + dwx;
Y34 = -t11 - t5;
Y35 = 0;
Y36 = 0;
Y37 = 0;
Y38 = 0;
Y39 = 0;
Y310 = 0;
Y311 = 0;
Y312 = 0;
Y313 = 0;
Y41 = 0;
Y42 = 0;
Y43 = Y31;
Y44 = -Y21;
Y45 = 0;
Y46 = Y33;
Y47 = -Y24;
Y48 = Y32;
Y49 = -Y22;
Y410 = -t5 + t6;
Y411 = dwx;
Y412 = -t12;
Y413 = t12;
Y51 = 0;
Y52 = -Y31;
Y53 = 0;
Y54 = Y11;
Y55 = -Y32;
Y56 = 0;
Y57 = Y14;
Y58 = -Y33;
Y59 = t11 - t6;
Y510 = Y13;
Y511 = t8;
Y512 = dwy;
Y513 = -t8;
Y61 = 0;
Y62 = Y21;
Y63 = -Y11;
Y64 = 0;
Y65 = Y22;
Y66 = -Y13;
Y67 = 0;
Y68 = t5 - t11;
Y69 = Y24;
Y610 = -Y14;
Y611 = -t7;
Y612 = t7;
Y613 = dwz;

YB42 = [Y11 Y12 Y13 Y14 Y15 Y16 Y17 Y18 Y19 Y110 Y111 Y112 Y113;...
        Y21 Y22 Y23 Y24 Y25 Y26 Y27 Y28 Y29 Y210 Y211 Y212 Y213;...
        Y31 Y32 Y33 Y34 Y35 Y36 Y37 Y38 Y39 Y310 Y311 Y312 Y313;...
        Y41 Y42 Y43 Y44 Y45 Y46 Y47 Y48 Y49 Y410 Y411 Y412 Y413;...
        Y51 Y52 Y53 Y54 Y55 Y56 Y57 Y58 Y59 Y510 Y511 Y512 Y513;...
        Y61 Y62 Y63 Y64 Y65 Y66 Y67 Y68 Y69 Y610 Y611 Y612 Y613];

== matlab function WMMSupportingForcesGP2020a/MATLAB Function3 ==
  data: GRotBC input; TRL_fz output; l1 parameter; l2 parameter; mw parameter; Rw parameter; zC parameter; mBC parameter; w parameter; BMF input; xCA parameter; yCA parameter; zCA parameter; BCvX input; BCvY input; dPsi input; BCaX input; BCaY input; ddPsi input; g0 parameter; BCI parameter size=[3,3]
function TRL_fz = fcn(GRotBC, l1, l2, mw, Rw, zC, mBC, w, BMF, xCA, yCA, zCA, BCvX, BCvY, dPsi, BCaX, BCaY, ddPsi, g0, BCI)


r31 = GRotBC(3,1); r32 = GRotBC(3,2); r33 = GRotBC(3,3);

BMfx = BMF(1);     BMfy = BMF(2);     BMfz = BMF(3);
BMmx = BMF(4);     BMmy = BMF(5);     

BCIxz = BCI(1,3);  BCIyz = BCI(2,3);

zetaRL1 = g0*(mBC/2 * l2/(l1+l2) + mw)*r33 - g0*(mw*Rw + 0.25*mBC*zC)/w*r32 +...
          2*g0*(mw*Rw + 0.25*mBC*zC)/(l1+l2)*r31;
zetaRL2 = -0.5*(zCA + zC)/(l1+l2)*BMfx;
zetaRL3 = 0.25*(zCA + zC)/w*BMfy;
zetaRL4 = -0.5*((l2-xCA)/(l1+l2) + 0.5*yCA/w)*BMfz;
zetaRL5 = -BMmx/4/w;
zetaRL6 = -0.5*BMmy/(l1+l2);
zetaRL7 = 0.5*mBC*zC/(l1+l2)*BCaX;
zetaRL8 = -0.25*mBC*zC/w*BCaY;
zetaRL9 = -0.5*mBC*zC*(BCvX/(2*w) + BCvY/(l1+l2))*dPsi;
zetaRL10 = 0.5*(BCIxz/(l1+l2) - BCIyz/(2*w))*dPsi*dPsi;
zetaRL11 = 0.5*(BCIyz/(l1+l2) + BCIxz/(2*w))*ddPsi;

TRL_fz = zetaRL1 + zetaRL2 + zetaRL3+ zetaRL4 + zetaRL5 + zetaRL6 + ...
         zetaRL7 + zetaRL8 + zetaRL9 + zetaRL10 + zetaRL11;

== matlab function WMMSupportingForcesGP2020a/calc_wheel_velocities_and_sideslip_angles_from_meas/Hydraulic manipulator, calculation/AnalyticTotalForces/Structure 1/MATLAB Function ==
  data: thetaBc1 output; Bc1_r_Bc1C parameter; mBc1 parameter; Bc1cI parameter
function thetaBc1 = thetaBc1(Bc1_r_Bc1C, mBc1, Bc1cI)

rx = Bc1_r_Bc1C(1);
ry = Bc1_r_Bc1C(2);
rz = Bc1_r_Bc1C(3);

Ixx = Bc1cI(1,1);
Iyy = Bc1cI(2,2);
Izz = Bc1cI(3,3);
Iyz = Bc1cI(2,3);
Ixz = Bc1cI(1,3);
Ixy = Bc1cI(1,2);

t1 = rx*rx;
t2 = ry*ry;
t3 = rz*rz;
t4 = rx*mBc1;

thetaBc1 = [mBc1; rx*mBc1; ry*mBc1; rz*mBc1; t1*mBc1; t2*mBc1; t3*mBc1; t4*ry - Ixy; t4*rz - Ixz; mBc1*ry*rz - Iyz; Ixx; Iyy; Izz];

== matlab function WMMSupportingForcesGP2020a/calc_wheel_velocities_and_sideslip_angles_from_meas/Hydraulic manipulator, calculation/AnalyticTotalForces/Structure 1/MATLAB Function1 ==
  data: Bc1V input; Bc1a input; Bc1w input; Bc1dw input; Bc1_Rot_W input; Wg parameter; YBc1 output
function YBc1  = thetaBc1(Bc1V, Bc1a, Bc1w, Bc1dw, Bc1_Rot_W,  Wg)

vx = Bc1V(1);
vy = Bc1V(2);
vz = Bc1V(3);
ax = Bc1a(1);
ay = Bc1a(2);
az = Bc1a(3);
wx = Bc1w(1);
wy = Bc1w(2);
wz = Bc1w(3);
dwx = Bc1dw(1);
dwy = Bc1dw(2);
dwz = Bc1dw(3);
Bc1g = Bc1_Rot_W*Wg;
gx = Bc1g(1);
gy = Bc1g(2);
gz = Bc1g(3);

Y11 = ( ax + vz * wy - vy * wz  + gx);
t5 = (wy *  wy);
t6 = (wz * wz);
Y12 = -t5 - t6;
t7 = (wx * wy);
Y13 = (t7 - dwz);
t8 = (wx * wz);
Y14 = (t8 + dwy);
Y15 = 0;
Y16 = 0;
Y17 = 0;
Y18 = 0;
Y19 = 0;
Y110 = 0;
Y111 = 0;
Y112 = 0;
Y113 = 0;
Y21 = vx * wz - vz * wx + ay + gy;
Y22 = t7 + dwz;
t11 = wx * wx;
Y23 = -t11 - t6;
t12 = wy * wz;
Y24 = t12 - dwx;
Y25 = 0;
Y26 = 0;
Y27 = 0;
Y28 = 0;
Y29 = 0;
Y210 = 0;
Y211 = 0;
Y212 = 0;
Y213 = 0;
Y31 = -vx * wy + vy * wx + az + gz;
Y32 = t8 - dwy;
Y33 = t12 + dwx;
Y34 = -t11 - t5;
Y35 = 0;
Y36 = 0;
Y37 = 0;
Y38 = 0;
Y39 = 0;
Y310 = 0;
Y311 = 0;
Y312 = 0;
Y313 = 0;
Y41 = 0;
Y42 = 0;
Y43 = Y31;
Y44 = -Y21;
Y45 = 0;
Y46 = Y33;
Y47 = -Y24;
Y48 = Y32;
Y49 = -Y22;
Y410 = -t5 + t6;
Y411 = dwx;
Y412 = -t12;
Y413 = t12;
Y51 = 0;
Y52 = -Y31;
Y53 = 0;
Y54 = Y11;
Y55 = -Y32;
Y56 = 0;
Y57 = Y14;
Y58 = -Y33;
Y59 = t11 - t6;
Y510 = Y13;
Y511 = t8;
Y512 = dwy;
Y513 = -t8;
Y61 = 0;
Y62 = Y21;
Y63 = -Y11;
Y64 = 0;
Y65 = Y22;
Y66 = -Y13;
Y67 = 0;
Y68 = t5 - t11;
Y69 = Y24;
Y610 = -Y14;
Y611 = -t7;
Y612 = t7;
Y613 = dwz;

YBc1 = [Y11 Y12 Y13 Y14 Y15 Y16 Y17 Y18 Y19 Y110 Y111 Y112 Y113;...
        Y21 Y22 Y23 Y24 Y25 Y26 Y27 Y28 Y29 Y210 Y211 Y212 Y213;...
        Y31 Y32 Y33 Y34 Y35 Y36 Y37 Y38 Y39 Y310 Y311 Y312 Y313;...
        Y41 Y42 Y43 Y44 Y45 Y46 Y47 Y48 Y49 Y410 Y411 Y412 Y413;...
        Y51 Y52 Y53 Y54 Y55 Y56 Y57 Y58 Y59 Y510 Y511 Y512 Y513;...
        Y61 Y62 Y63 Y64 Y65 Y66 Y67 Y68 Y69 Y610 Y611 Y612 Y613];

== matlab function WMMSupportingForcesGP2020a/calc_wheel_velocities_and_sideslip_angles_from_meas/Hydraulic manipulator, calculation/AnalyticVelocities/Structure 1/GeomPropS1/Subsystem/LiftPistonVelocity ==
  data: dq1 input; x1 input; q1 input; dx1 output; L1 parameter; L11 parameter; x10 parameter
function dx1 = dx1(dq1, x1, q1, L1, L11, x10)

dx1 = -(L1*L11*sin(q1))/(x1+x10)*dq1;

== matlab function WMMSupportingForcesGP2020a/Mobile Manipulator in Simscape/WFR_kinematic_quantities/lateralForceFR ==
  data: FzFR input; alphaFR input; FyFR output
function FyFR = latForceFR(FzFR, alphaFR)

Dy = 0.5;
Ey = -0.9;
By = -11.37;
Cy = 1.33;

FyFR = Dy*FzFR*sin(Cy*atan(By*alphaFR - Ey*(By*alphaFR - atan(By*alphaFR))));
